simulink model "gm_sampleModel2044_sub"  (R2023a)
settings: Solver=VariableStepAuto  StartTime=0.0  StopTime=10.0  RelTol=1e-3
libraries: hdlsllib x1
settings Model: Creator=user1  LastModifiedBy=user1
settings OptimizationCC: BlockReduction=off  ConditionallyExecuteInputs=off
settings DebuggingCC: InheritedTsInSrcMsg=none

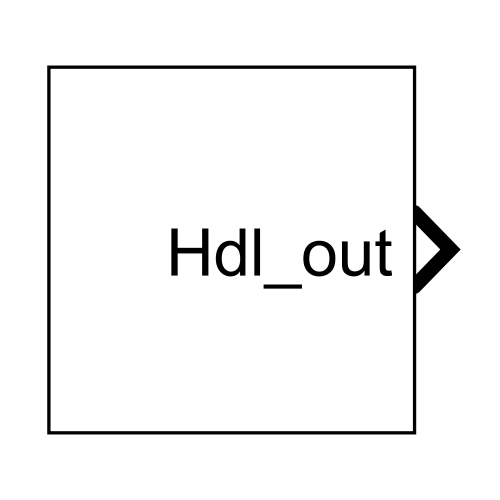
[thumbnail: Simulink's stored preview of the top-level diagram]
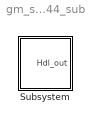
== system gm_sampleModel2044_sub ==
  Subsystem : Subsystem

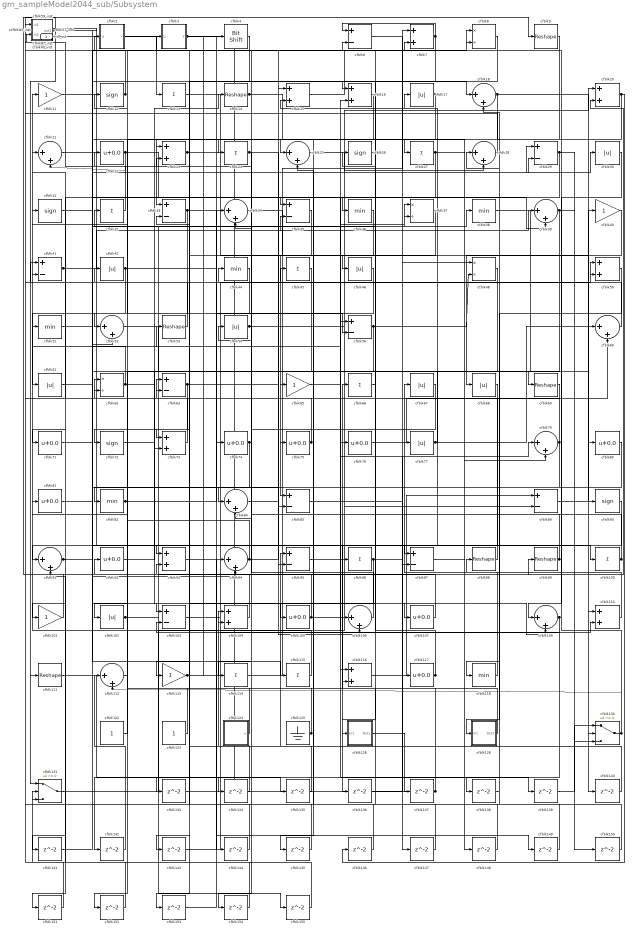
== system gm_sampleModel2044_sub/Subsystem ==
  cfblk1 : Constant  Value=0  OutDataTypeStr=uint8  SampleTime=1
  cfblk{13,24,27,32,45,66,96,100,114..115} (10 alike) : Sum  Inputs=+  OutDataTypeStr=uint8
  cfblk{11,40,65,101,113} (5 alike) : Gain  OutDataTypeStr=uint8
  cfblk{17,30,42,46,54,61,67..68,77,102} (10 alike) : Abs  OutDataTypeStr=uint8  SaturateOnIntegerOverflow=off
  cfblk{6,29,33,35,41,56,63,85,89,95,97,103} (12 alike) : Sum  Inputs=+-  OutDataTypeStr=uint8
  cfblk{7,15..16,20,23,50,73,93,104,110,116} (11 alike) : Sum  OutDataTypeStr=uint8
  cfblk{22,71,74..76,80..81,92,105,107,117} (11 alike) : Bias  Bias=0.0  SaturateOnIntegerOverflow=off
  cfblk{18,21,25,28,34,39,52,60,79,84,91,94,106,109,112} (15 alike) : Sum  Inputs=|++  OutDataTypeStr=uint8
  cfblk108_inst : Subsystem
  cfblk{9,14,53,69,98..99,111} (7 alike) : Reshape
  cfblk{36,38,44,51,82,118} (6 alike) : MinMax  OutDataTypeStr=uint8
  cfblk{12,26,31,72,90} (5 alike) : Signum
  cfblk122 : Constant  OutDataTypeStr=uint8  SampleTime=-1
  cfblk123 : Constant  OutDataTypeStr=uint8  SampleTime=-1
  cfblk124 : Subsystem  mask(Counter Free-Running){NumBits=double(16), tsamp=double(-1)}
      mask prompts: NumBits "Simulink:masks:NumberOfBits_MP"; tsamp "Simulink:masks:SampleTime_MP"
      mask help: Simulink:masks:CounterFreeRunning_MD
  cfblk125 : Ground
  cfblk126 : Subsystem
  cfblk128 : Subsystem
  cfblk130 : Switch  OutDataTypeStr=uint8  SaturateOnIntegerOverflow=off  InputSameDT=off
  cfblk131 : Switch  OutDataTypeStr=uint8  SaturateOnIntegerOverflow=off  InputSameDT=off
  cfblk{133..155} (23 alike) : Delay  SampleTime=1
  cfblk19_inst : Subsystem
  cfblk2 : Subsystem  mask(Detect Fall Nonpositive){vinit=double(0), InputProcessing=Elements as channels (sample based), OutDataTypeStr=uint8}
      mask prompts: vinit "Simulink:masks:InitialCondition_MP"; InputProcessing "Simulink:masks:InputProcessing_MP"; OutDataTypeStr "Simulink:masks:OutputDataType_MP"
      mask help: Simulink:masks:DetectFallNonpositive_MD
      mask init:
      | InputProcessing = 'Elements as channels (sample based)';
      | OutDataTypeStr = 'uint8';
      | vinit = double(0);
      mask TypeOptions InputProcessing: Simulink:masks:ColumnsAsChannelsFrameBased | Simulink:masks:ElementsAsChannelsSampleBased
      mask TypeOptions OutDataTypeStr: Simulink:masks:uint8 | Simulink:masks:boolean
      mask Display: fprintf('U <= 0\n&  NOT\nU/z <= 0')
  cfblk3 : Subsystem  mask(Detect Fall Negative){vinit=double(0), InputProcessing=Elements as channels (sample based), OutDataTypeStr=uint8}
      mask prompts: vinit "Simulink:masks:InitialCondition_MP"; InputProcessing "Simulink:masks:InputProcessing_MP"; OutDataTypeStr "Simulink:masks:OutputDataType_MP"
      mask help: Simulink:masks:DetectFallNegative_MD
      mask init:
      | InputProcessing = 'Elements as channels (sample based)';
      | OutDataTypeStr = 'uint8';
      | vinit = double(0);
      mask TypeOptions InputProcessing: Simulink:masks:ColumnsAsChannelsFrameBased | Simulink:masks:ElementsAsChannelsSampleBased
      mask TypeOptions OutDataTypeStr: Simulink:masks:uint8 | Simulink:masks:boolean
      mask Display: fprintf('U < 0\n&  NOT\nU/z < 0')
  cfblk{8,37,48,62} (4 alike) : Product  Inputs=*/  OutDataTypeStr=uint8  RndMeth=Zero  SaturateOnIntegerOverflow=on
  cfblk4 : hdlsllib/Logic and Bit Operations/Bit Shift  mode=Shift Left Logical  N=0
  cfblk43_inst : Subsystem
  cfblk47_inst : Subsystem
  cfblk57_inst : Subsystem
  cfblk59_inst : Subsystem
  cfblk83_inst : Subsystem
  cfblk87_inst : Subsystem
  Hdl_out : Outport  OutDataTypeStr=uint8  SampleTime=1
  wires:
  cfblk1/1 -> cfblk25/1
  cfblk100/1 -> cfblk57_inst/2(in2), cfblk44/1
  cfblk101/1 -> cfblk9/1
  cfblk102/1 -> cfblk20/2, cfblk155/1, cfblk38/1
  cfblk103/1 -> cfblk50/1
  cfblk104/1 -> cfblk83_inst/1(in1)
  cfblk105/1 -> cfblk93/2, cfblk20/1
  cfblk106/1 -> cfblk108_inst/1(in1)
  cfblk107/1 -> cfblk92/1
  cfblk108_inst/1(out1) -> cfblk27/1
  cfblk109/1 -> cfblk103/2, cfblk142/1
  cfblk11/1 -> cfblk136/1
  cfblk110/1 -> cfblk67/1
  cfblk111/1 -> cfblk135/1
  cfblk112/1 -> cfblk12/1
  cfblk113/1 -> cfblk99/1, cfblk4/1, cfblk110/2
  cfblk114/1 -> cfblk7/1
  cfblk115/1 -> cfblk11/1
  cfblk116/1 -> cfblk89/1
  cfblk117/1 -> cfblk6/2, cfblk32/1
  cfblk118/1 -> cfblk98/1
  cfblk12/1 -> cfblk87_inst/2(in2), cfblk19_inst/1(in1)
  cfblk122/1 -> cfblk62/1
  cfblk123/1 -> cfblk81/1
  cfblk124/1(y) -> cfblk31/1
  cfblk125/1 -> cfblk43_inst/2(in2), cfblk108_inst/2(in2)
  cfblk126/1(Out1) -> cfblk137/1
  cfblk128/1(Out1) -> cfblk66/1
  cfblk13/1 -> cfblk85/1
  cfblk130/1 -> cfblk112/2, cfblk2/1(U), cfblk45/1
  cfblk131/1 -> cfblk104/1
  cfblk133/1 -> cfblk89/2
  cfblk134/1 -> cfblk33/2
  cfblk135/1 -> cfblk104/2
  cfblk136/1 -> cfblk79/1
  cfblk137/1 -> cfblk41/2, Hdl_out/1
  cfblk138/1 -> cfblk18/2
  cfblk139/1 -> cfblk130/1
  cfblk14/1 -> cfblk148/1, cfblk147/1
  cfblk140/1 -> cfblk95/1
  cfblk141/1 -> cfblk37/1
  cfblk142/1 -> cfblk112/1
  cfblk143/1 -> cfblk16/2
  cfblk144/1 -> cfblk63/1
  cfblk145/1 -> cfblk47_inst/2(in2)
  cfblk146/1 -> cfblk25/2
  cfblk147/1 -> cfblk19_inst/2(in2)
  cfblk148/1 -> cfblk116/2
  cfblk149/1 -> cfblk28/1
  cfblk15/1 -> cfblk7/2
  cfblk150/1 -> cfblk59_inst/2(in2)
  cfblk151/1 -> cfblk131/2
  cfblk152/1 -> cfblk131/3
  cfblk153/1 -> cfblk94/1
  cfblk154/1 -> cfblk83_inst/2(in2)
  cfblk155/1 -> cfblk91/2
  cfblk16/1 -> cfblk33/1
  cfblk17/1 -> cfblk52/1, cfblk35/1, cfblk15/2
  cfblk18/1 -> cfblk90/1, cfblk65/1
  cfblk19_inst/1(out1) -> cfblk69/1, cfblk111/1
  cfblk2/1(Y) -> cfblk13/1
  cfblk20/1 -> cfblk146/1, cfblk145/1
  cfblk21/1 -> cfblk74/1
  cfblk22/1 -> cfblk76/1, cfblk21/2
  cfblk23/1 -> cfblk140/1, cfblk96/1
  cfblk24/1 -> cfblk34/2, cfblk106/2
  cfblk25/1 -> cfblk28/2
  cfblk26/1 -> cfblk126/1(In1)
  cfblk27/1 -> cfblk84/2, cfblk79/2
  cfblk28/1 -> cfblk47_inst/1(in1)
  cfblk29/1 -> cfblk75/1, cfblk71/1, cfblk150/1
  cfblk3/1(Y) -> cfblk95/2, cfblk149/1
  cfblk30/1 -> cfblk109/1
  cfblk31/1 -> cfblk29/2
  cfblk32/1 -> cfblk43_inst/1(in1)
  cfblk33/1 -> cfblk61/1, cfblk116/1
  cfblk34/1 -> cfblk80/1
  cfblk35/1 -> cfblk113/1
  cfblk36/1 -> cfblk73/1
  cfblk37/1 -> cfblk46/1
  cfblk38/1 -> cfblk130/2
  cfblk39/1 -> cfblk73/2, cfblk130/3, cfblk82/1
  cfblk4/1 -> cfblk93/1
  cfblk40/1 -> cfblk68/1
  cfblk41/1 -> cfblk52/2, cfblk39/1
  cfblk42/1 -> cfblk56/2, cfblk151/1
  cfblk43_inst/1(out1) -> cfblk84/1, cfblk100/1
  cfblk44/1 -> cfblk141/1
  cfblk45/1 -> cfblk134/1
  cfblk46/1 -> cfblk91/1
  cfblk47_inst/1(out1) -> cfblk39/2, cfblk131/1
  cfblk48/1 -> cfblk97/1
  cfblk50/1 -> cfblk128/1(In1)
  cfblk51/1 -> cfblk29/1
  cfblk52/1 -> cfblk110/1
  cfblk53/1 -> cfblk41/1
  cfblk54/1 -> cfblk50/2, cfblk138/1
  cfblk56/1 -> cfblk48/2, cfblk152/1
  cfblk57_inst/1(out1) -> cfblk115/1
  cfblk59_inst/1(out1) -> cfblk87_inst/1(in1), cfblk18/1
  cfblk6/1 -> cfblk48/1
  cfblk60/1 -> cfblk57_inst/1(in1)
  cfblk61/1 -> cfblk8/1
  cfblk62/1 -> cfblk35/2, cfblk51/1
  cfblk63/1 -> cfblk72/1, cfblk15/1
  cfblk65/1 -> cfblk37/2
  cfblk66/1 -> cfblk26/1
  cfblk67/1 -> cfblk114/1
  cfblk68/1 -> cfblk106/1
  cfblk69/1 -> cfblk62/2
  cfblk7/1 -> cfblk6/1, cfblk23/1
  cfblk71/1 -> cfblk94/2
  cfblk72/1 -> cfblk107/1
  cfblk73/1 -> cfblk22/1
  cfblk74/1 -> cfblk154/1, cfblk153/1
  cfblk75/1 -> cfblk23/2, cfblk3/1(U)
  cfblk76/1 -> cfblk60/2
  cfblk77/1 -> cfblk60/1, cfblk17/1
  cfblk79/1 -> cfblk21/1, cfblk118/1
  cfblk8/1 -> cfblk36/1
  cfblk80/1 -> cfblk102/1
  cfblk81/1 -> cfblk85/2
  cfblk82/1 -> cfblk34/1, cfblk109/2
  cfblk83_inst/1(out1) -> cfblk16/1, cfblk24/1
  cfblk84/1 -> cfblk30/1
  cfblk85/1 -> cfblk97/2
  cfblk87_inst/1(out1) -> cfblk103/1
  cfblk89/1 -> cfblk40/1
  cfblk9/1 -> cfblk133/1
  cfblk90/1 -> cfblk101/1
  cfblk91/1 -> cfblk56/1, cfblk53/1
  cfblk92/1 -> cfblk14/1
  cfblk93/1 -> cfblk144/1
  cfblk94/1 -> cfblk42/1, cfblk8/2
  cfblk95/1 -> cfblk77/1
  cfblk96/1 -> cfblk117/1, cfblk105/1, cfblk143/1
  cfblk97/1 -> cfblk139/1
  cfblk98/1 -> cfblk59_inst/1(in1)
  cfblk99/1 -> cfblk63/2, cfblk54/1

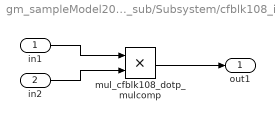
== system gm_sampleModel2044_sub/Subsystem/cfblk108_inst ==
  in1 : Inport  OutDataTypeStr=uint8  SampleTime=1
  in2 : Inport  Port=2  OutDataTypeStr=uint8  SampleTime=1
  mul_cfblk108_dotp_mulcomp : Product  Inputs=**  OutDataTypeStr=uint8  SampleTime=1
  out1 : Outport  OutDataTypeStr=uint8  SampleTime=1
  wires:
  in1/1 -> mul_cfblk108_dotp_mulcomp/1
  in2/1 -> mul_cfblk108_dotp_mulcomp/2
  mul_cfblk108_dotp_mulcomp/1 -> out1/1

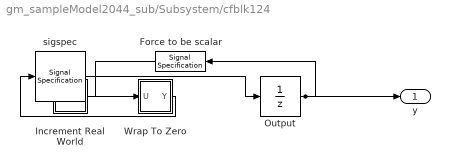
== system gm_sampleModel2044_sub/Subsystem/cfblk124 ==
  Force to be scalar : SignalSpecification  DisableCoverage=on  Dimensions=1
  Increment Real World : Subsystem  mask(Real World Value Increment){}
      mask help: Simulink:masks:RealWorldValueIncrement_MD
      mask Display: disp('V++')
  Output : UnitDelay  InitialCondition=0.0  SampleTime=tsamp  HasFrameUpgradeWarning=on
  Wrap To Zero : Subsystem  mask(Wrap To Zero){Threshold=double(65535)}
      mask prompts: Threshold "Simulink:masks:Threshold_MP"
      mask help: Simulink:masks:WrapToZero_MD
  sigspec : SignalSpecification  OutDataTypeStr=uint16  Dimensions=1
  y : Outport  SampleTime=1
  wires:
  Force to be scalar/1 -> Increment Real World/1(u)
  Increment Real World/1(y) -> Wrap To Zero/1(U)
  Output/1 -> Force to be scalar/1, y/1
  Wrap To Zero/1(Y) -> sigspec/1
  sigspec/1 -> Output/1

== system gm_sampleModel2044_sub/Subsystem/cfblk126 ==
  In1 : Inport  OutDataTypeStr=uint8  PortDimensions=1  SampleTime=1
  Out1 : Outport  SampleTime=1
  wires:
  In1/1 -> Out1/1

== system gm_sampleModel2044_sub/Subsystem/cfblk128 ==
  In1 : Inport  OutDataTypeStr=uint8  PortDimensions=1  SampleTime=1
  Out1 : Outport  SampleTime=1
  wires:
  In1/1 -> Out1/1

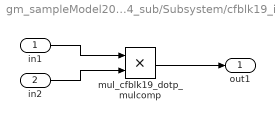
== system gm_sampleModel2044_sub/Subsystem/cfblk19_inst ==
  in1 : Inport  OutDataTypeStr=uint8  SampleTime=1
  in2 : Inport  Port=2  OutDataTypeStr=uint8  SampleTime=1
  mul_cfblk19_dotp_mulcomp : Product  Inputs=**  OutDataTypeStr=uint8  SampleTime=1
  out1 : Outport  OutDataTypeStr=uint8  SampleTime=1
  wires:
  in1/1 -> mul_cfblk19_dotp_mulcomp/1
  in2/1 -> mul_cfblk19_dotp_mulcomp/2
  mul_cfblk19_dotp_mulcomp/1 -> out1/1

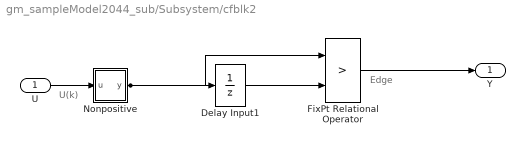
== system gm_sampleModel2044_sub/Subsystem/cfblk2 ==
  note: U(k)
  note: Edge
  U : Inport  OutDataTypeStr=uint8  SampleTime=1
  Delay Input1 : UnitDelay  Description=Store in Global RAM  DisableCoverage=on  InitialCondition=vinit  SampleTime=-1  HasFrameUpgradeWarning=on
  FixPt Relational Operator : RelationalOperator  Operator=>  OutDataTypeStr=fixdt(0, 8)  ZeroCross=off  InputSameDT=off
  Nonpositive : Subsystem  mask(Compare To Zero){relop=<=, OutDataTypeStr=boolean, ZeroCross=off}
      mask prompts: relop "Simulink:masks:Operator_MP"; OutDataTypeStr "Simulink:masks:OutputDataType_MP"; ZeroCross "Simulink:masks:EnableZerocrossingDetection_MP"
      mask help: Simulink:masks:CompareToZero_MD
      mask init:
      | OutDataTypeStr = 'boolean';
      | ZeroCross = 'off';
      | blkName = 'sampleModel2044_sub/Subsystem/cfblk2/Nonpositive';
      | relop = '<=';
      | setValue = 'boolean';
      mask TypeOptions relop: == | ~= | < | <= | >= | >
      mask TypeOptions OutDataTypeStr: Simulink:masks:uint8 | Simulink:masks:boolean
      mask Callback ZeroCross: sl('zeroCrossEnable', gcbh);
      mask Display: disp([relop,' 0'])
  Y : Outport  SampleTime=1
  wires:
  U/1 -> Nonpositive/1(u)
  Delay Input1/1 -> FixPt Relational Operator/2
  FixPt Relational Operator/1 -> Y/1
  Nonpositive/1(y) -> FixPt Relational Operator/1, Delay Input1/1

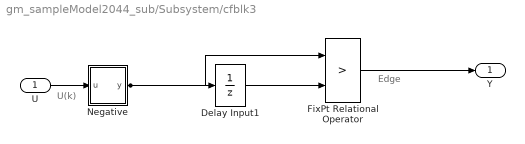
== system gm_sampleModel2044_sub/Subsystem/cfblk3 ==
  note: U(k)
  note: Edge
  U : Inport  OutDataTypeStr=uint8  SampleTime=1
  Delay Input1 : UnitDelay  Description=Store in Global RAM  DisableCoverage=on  InitialCondition=vinit  SampleTime=-1  HasFrameUpgradeWarning=on
  FixPt Relational Operator : RelationalOperator  Operator=>  OutDataTypeStr=fixdt(0, 8)  ZeroCross=off  InputSameDT=off
  Negative : Subsystem  mask(Compare To Zero){relop=<, OutDataTypeStr=boolean, ZeroCross=off}
      mask prompts: relop "Simulink:masks:Operator_MP"; OutDataTypeStr "Simulink:masks:OutputDataType_MP"; ZeroCross "Simulink:masks:EnableZerocrossingDetection_MP"
      mask help: Simulink:masks:CompareToZero_MD
      mask init:
      | OutDataTypeStr = 'boolean';
      | ZeroCross = 'off';
      | blkName = 'sampleModel2044_sub/Subsystem/cfblk3/Negative';
      | relop = '<';
      | setValue = 'boolean';
      mask TypeOptions relop: == | ~= | < | <= | >= | >
      mask TypeOptions OutDataTypeStr: Simulink:masks:uint8 | Simulink:masks:boolean
      mask Callback ZeroCross: sl('zeroCrossEnable', gcbh);
      mask Display: disp([relop,' 0'])
  Y : Outport  SampleTime=1
  wires:
  U/1 -> Negative/1(u)
  Delay Input1/1 -> FixPt Relational Operator/2
  FixPt Relational Operator/1 -> Y/1
  Negative/1(y) -> FixPt Relational Operator/1, Delay Input1/1

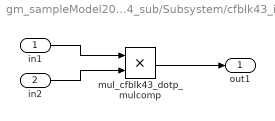
== system gm_sampleModel2044_sub/Subsystem/cfblk43_inst ==
  in1 : Inport  OutDataTypeStr=uint8  SampleTime=1
  in2 : Inport  Port=2  OutDataTypeStr=uint8  SampleTime=1
  mul_cfblk43_dotp_mulcomp : Product  Inputs=**  OutDataTypeStr=uint8  SampleTime=1
  out1 : Outport  OutDataTypeStr=uint8  SampleTime=1
  wires:
  in1/1 -> mul_cfblk43_dotp_mulcomp/1
  in2/1 -> mul_cfblk43_dotp_mulcomp/2
  mul_cfblk43_dotp_mulcomp/1 -> out1/1

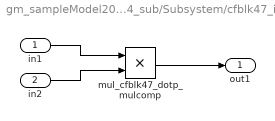
== system gm_sampleModel2044_sub/Subsystem/cfblk47_inst ==
  in1 : Inport  OutDataTypeStr=uint8  SampleTime=1
  in2 : Inport  Port=2  OutDataTypeStr=uint8  SampleTime=1
  mul_cfblk47_dotp_mulcomp : Product  Inputs=**  OutDataTypeStr=uint8  SampleTime=1
  out1 : Outport  OutDataTypeStr=uint8  SampleTime=1
  wires:
  in1/1 -> mul_cfblk47_dotp_mulcomp/1
  in2/1 -> mul_cfblk47_dotp_mulcomp/2
  mul_cfblk47_dotp_mulcomp/1 -> out1/1

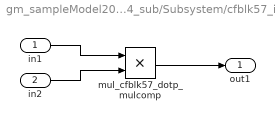
== system gm_sampleModel2044_sub/Subsystem/cfblk57_inst ==
  in1 : Inport  OutDataTypeStr=uint8  SampleTime=1
  in2 : Inport  Port=2  OutDataTypeStr=uint8  SampleTime=1
  mul_cfblk57_dotp_mulcomp : Product  Inputs=**  OutDataTypeStr=uint8  SampleTime=1
  out1 : Outport  OutDataTypeStr=uint8  SampleTime=1
  wires:
  in1/1 -> mul_cfblk57_dotp_mulcomp/1
  in2/1 -> mul_cfblk57_dotp_mulcomp/2
  mul_cfblk57_dotp_mulcomp/1 -> out1/1

== system gm_sampleModel2044_sub/Subsystem/cfblk59_inst ==
  in1 : Inport  OutDataTypeStr=uint8  SampleTime=1
  in2 : Inport  Port=2  OutDataTypeStr=uint8  SampleTime=1
  mul_cfblk59_dotp_mulcomp : Product  Inputs=**  OutDataTypeStr=uint8  SampleTime=1
  out1 : Outport  OutDataTypeStr=uint8  SampleTime=1
  wires:
  in1/1 -> mul_cfblk59_dotp_mulcomp/1
  in2/1 -> mul_cfblk59_dotp_mulcomp/2
  mul_cfblk59_dotp_mulcomp/1 -> out1/1

== system gm_sampleModel2044_sub/Subsystem/cfblk83_inst ==
  in1 : Inport  OutDataTypeStr=uint8  SampleTime=1
  in2 : Inport  Port=2  OutDataTypeStr=uint8  SampleTime=1
  mul_cfblk83_dotp_mulcomp : Product  Inputs=**  OutDataTypeStr=uint8  SampleTime=1
  out1 : Outport  OutDataTypeStr=uint8  SampleTime=1
  wires:
  in1/1 -> mul_cfblk83_dotp_mulcomp/1
  in2/1 -> mul_cfblk83_dotp_mulcomp/2
  mul_cfblk83_dotp_mulcomp/1 -> out1/1

== system gm_sampleModel2044_sub/Subsystem/cfblk87_inst ==
  in1 : Inport  OutDataTypeStr=uint8  SampleTime=1
  in2 : Inport  Port=2  OutDataTypeStr=uint8  SampleTime=1
  mul_cfblk87_dotp_mulcomp : Product  Inputs=**  OutDataTypeStr=uint8  SampleTime=1
  out1 : Outport  OutDataTypeStr=uint8  SampleTime=1
  wires:
  in1/1 -> mul_cfblk87_dotp_mulcomp/1
  in2/1 -> mul_cfblk87_dotp_mulcomp/2
  mul_cfblk87_dotp_mulcomp/1 -> out1/1

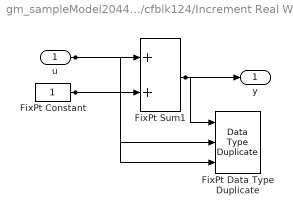
== system gm_sampleModel2044_sub/Subsystem/cfblk124/Increment Real World ==
  u : Inport  OutDataTypeStr=uint16  SampleTime=1
  FixPt Constant : Constant  DisableCoverage=on  OutDataTypeStr=Inherit: Inherit via back propagation  SampleTime=-1
  FixPt Data Type Duplicate : DataTypeDuplicate  DisableCoverage=on  NumInputPorts=3
  FixPt Sum1 : Sum  InputSameDT=on  OutDataTypeStr=Inherit: Inherit via back propagation  LockScale=on
  y : Outport  SampleTime=1
  wires:
  u/1 -> FixPt Sum1/1, FixPt Data Type Duplicate/2
  FixPt Constant/1 -> FixPt Sum1/2, FixPt Data Type Duplicate/3
  FixPt Sum1/1 -> FixPt Data Type Duplicate/1, y/1

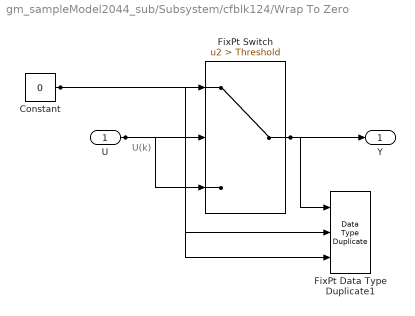
== system gm_sampleModel2044_sub/Subsystem/cfblk124/Wrap To Zero ==
  note: U(k)
  U : Inport  OutDataTypeStr=uint16  SampleTime=1
  Constant : Constant  DisableCoverage=on  Value=0  OutDataTypeStr=Inherit: Inherit via back propagation  SampleTime=-1
  FixPt Data Type Duplicate1 : DataTypeDuplicate  DisableCoverage=on  NumInputPorts=3
  FixPt Switch : Switch  Criteria=u2 > Threshold  Threshold=Threshold  OutDataTypeStr=Inherit: Inherit via back propagation  ZeroCross=off  SaturateOnIntegerOverflow=off  InputSameDT=off
  Y : Outport  SampleTime=1
  wires:
  U/1 -> FixPt Switch/3, FixPt Switch/2, FixPt Data Type Duplicate1/2
  Constant/1 -> FixPt Switch/1, FixPt Data Type Duplicate1/3
  FixPt Switch/1 -> FixPt Data Type Duplicate1/1, Y/1

== system gm_sampleModel2044_sub/Subsystem/cfblk2/Nonpositive ==
  u : Inport  OutDataTypeStr=uint8  SampleTime=1
  Compare : RelationalOperator  Operator=<=  OutDataTypeStr=boolean  ZeroCross=off
  Constant : Constant  DisableCoverage=on  Value=0  OutDataTypeStr=Inherit: Inherit via back propagation  SampleTime=-1  PreserveConstantTs=on
  y : Outport  SampleTime=1
  wires:
  u/1 -> Compare/1
  Compare/1 -> y/1
  Constant/1 -> Compare/2

== system gm_sampleModel2044_sub/Subsystem/cfblk3/Negative ==
  u : Inport  OutDataTypeStr=uint8  SampleTime=1
  Compare : RelationalOperator  Operator=<  OutDataTypeStr=boolean  ZeroCross=off
  Constant : Constant  DisableCoverage=on  Value=0  OutDataTypeStr=Inherit: Inherit via back propagation  SampleTime=-1  PreserveConstantTs=on
  y : Outport  SampleTime=1
  wires:
  u/1 -> Compare/1
  Compare/1 -> y/1
  Constant/1 -> Compare/2
